simulink model "a3e2"  (R2020a)
settings: Solver=FixedStepAuto  StartTime=0.0  StopTime=40000  FixedStep=0.01  RelTol=1e-3
undefined symbols (not defined in the file): DiscIntNeverNeededParam
libraries: sldvlib x17
settings Model: EnablePacing=on  PacingRate=2  Creator=mumun  LastModifiedBy=mumun
settings ConfigComp: DVMode=PropertyProving  DVMaxProcessTime=10000000000  DVTestSuiteOptimization=Auto  DVDetectOutOfBounds=on

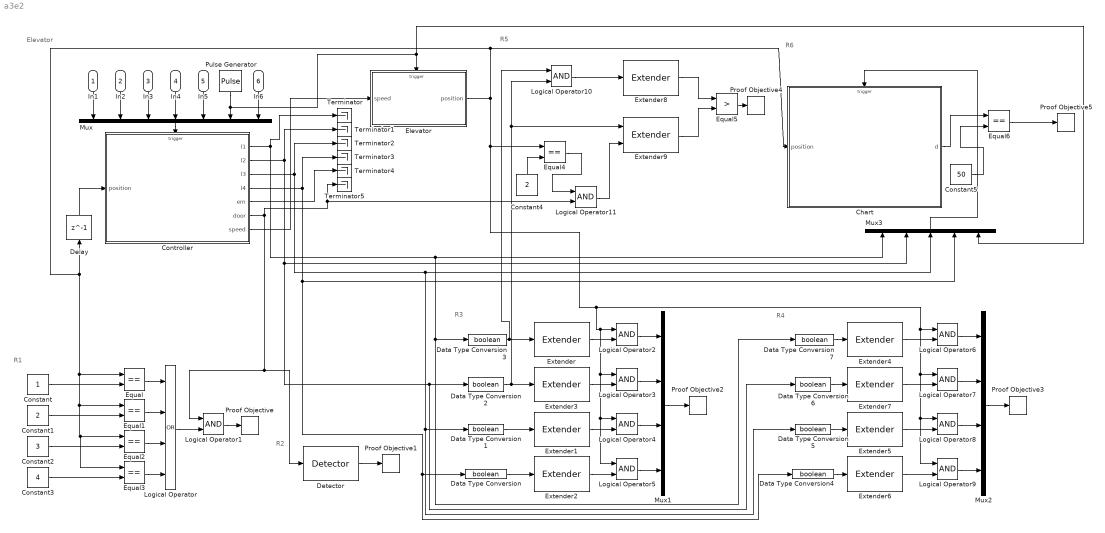
== system a3e2 ==
  note: R6
  note: R5
  note: R4
  note: Elevator
  note: R3
  note: R2
  note: R1
  In1 : Inport
  In2 : Inport  Port=2
  In3 : Inport  Port=3
  In4 : Inport  Port=4
  In5 : Inport  Port=5
  In6 : Inport  Port=6
  Chart : Stateflow chart  TreatAsAtomicUnit=on
  Constant : Constant
  Constant1 : Constant  Value=2
  Constant2 : Constant  Value=3
  Constant3 : Constant  Value=4
  Constant4 : Constant  Value=2
  Constant5 : Constant  Value=50
  Controller : Stateflow chart  TreatAsAtomicUnit=on
  Data Type Conversion{,1..7} (8 alike) : DataTypeConversion  OutDataTypeStr=boolean
  Delay : Delay  DelayLength=1  DelayLengthUpperLimit=2  InputProcessing=Columns as channels (frame based)  SampleTime=1
  Detector : sldvlib/Temporal Operators/Detector  reset=off  typ=Synchronized  in_hold=5  delay=1  out_hold=3
      settings: SourceProductBaseCode=SL
  Elevator : Stateflow chart  TreatAsAtomicUnit=on
  Equal{,1..4,6} (6 alike) : RelationalOperator  Operator===  OutDataTypeStr=boolean  RndMeth=Simplest
  Equal5 : RelationalOperator  Operator=>  OutDataTypeStr=boolean  RndMeth=Simplest
  Extender{,1..3} (4 alike) : sldvlib/Temporal Operators/Extender  reset=off  ext_type=Infinite  out_hold=5
      settings: SourceProductBaseCode=SL
  Extender{4..7} (4 alike) : sldvlib/Temporal Operators/Extender  reset=off  ext_type=Finite  out_hold=5
      settings: SourceProductBaseCode=SL
  Extender8 : sldvlib/Temporal Operators/Extender  reset=off  ext_type=Infinite  out_hold=3
      settings: SourceProductBaseCode=SL
  Extender9 : sldvlib/Temporal Operators/Extender  reset=on  ext_type=Infinite  out_hold=3
      settings: SourceProductBaseCode=SL
  Logical Operator : Logic  Operator=OR  Inputs=4  AllPortsSameDT=off  OutDataTypeStr=boolean
  Logical Operator{1..11} (11 alike) : Logic  AllPortsSameDT=off  OutDataTypeStr=boolean
  Mux : Mux  Inputs=7
  Mux1 : Mux
  Mux2 : Mux
  Mux3 : Mux  Inputs=5
  Proof Objective{,1..5} (6 alike) : sldvlib/Objectives and Constraints/Proof Objective  enabled=on  customAVTBlockType=Proof Objective  intervals=true  dispValues=on  outEnabled=off  enableStopSim=off
      settings: AttributesFormatString=%<intervals>  SourceProductBaseCode=SL
  Pulse Generator : DiscretePulseGenerator  PulseType=Time based  Period=1  PulseWidth=99  PhaseDelay=1
  Terminator{,1..5} (6 alike) : Terminator
  wires:
  In1/1 -> Mux/1
  In2/1 -> Mux/2
  In3/1 -> Mux/3
  In4/1 -> Mux/4
  In5/1 -> Mux/5
  Pulse Generator/1 -> Elevator/Trigger, Mux3/5, Mux/6
  Mux/1 -> Controller/Trigger
  In6/1 -> Mux/7
  Controller/5(em) -> Terminator4/1
  Controller/7(speed) -> Elevator/1(speed)
  Delay/1 -> Controller/1(position)
  Controller/1(l1) -> Terminator/1, Mux3/1, Data Type Conversion3/1, Data Type Conversion7/1
  Controller/2(l2) -> Terminator1/1, Mux3/2, Data Type Conversion6/1, Data Type Conversion2/1
  Controller/3(l3) -> Terminator2/1, Mux3/3, Data Type Conversion5/1, Data Type Conversion1/1
  Controller/4(l4) -> Terminator3/1, Mux3/4, Data Type Conversion4/1, Data Type Conversion/1
  Controller/6(door) -> Logical Operator11/2, Terminator5/1, Logical Operator1/1, Detector/1
  Detector/1 -> Proof Objective1/1
  Extender/1 -> Logical Operator2/2
  Extender1/1 -> Logical Operator4/2
  Extender3/1 -> Logical Operator3/2
  Extender2/1 -> Logical Operator5/2
  Logical Operator2/1 -> Mux1/1
  Logical Operator3/1 -> Mux1/2
  Logical Operator4/1 -> Mux1/3
  Logical Operator5/1 -> Mux1/4
  Mux1/1 -> Proof Objective2/1
  Data Type Conversion/1 -> Extender2/1
  Data Type Conversion1/1 -> Extender1/1
  Data Type Conversion2/1 -> Extender3/1, Extender9/1, Logical Operator10/2
  Data Type Conversion3/1 -> Logical Operator10/1, Extender/1
  Constant/1 -> Equal/2
  Constant1/1 -> Equal1/2
  Constant3/1 -> Equal3/2
  Constant2/1 -> Equal2/2
  Equal/1 -> Logical Operator/1
  Equal1/1 -> Logical Operator/2
  Equal2/1 -> Logical Operator/3
  Equal3/1 -> Logical Operator/4
  Logical Operator/1 -> Logical Operator1/2
  Logical Operator1/1 -> Proof Objective/1
  Extender5/1 -> Logical Operator8/2
  Extender4/1 -> Logical Operator6/2
  Data Type Conversion7/1 -> Extender4/1
  Logical Operator9/1 -> Mux2/4
  Logical Operator8/1 -> Mux2/3
  Mux2/1 -> Proof Objective3/1
  Logical Operator6/1 -> Mux2/1
  Extender7/1 -> Logical Operator7/2
  Data Type Conversion6/1 -> Extender7/1
  Data Type Conversion5/1 -> Extender5/1
  Elevator/1(position) -> Equal3/1, Equal2/1, Equal1/1, Equal/1, Delay/1, Chart/1(position), Logical Operator5/1, Logical Operator4/1, Logical Operator3/1, Logical Operator2/1, Logical Operator9/1, Logical Operator8/1, Logical Operator7/1, Logical Operator6/1, Equal4/1
  Logical Operator7/1 -> Mux2/2
  Extender6/1 -> Logical Operator9/2
  Data Type Conversion4/1 -> Extender6/1
  Logical Operator10/1 -> Extender8/1
  Constant4/1 -> Equal4/2
  Equal4/1 -> Logical Operator11/1
  Logical Operator11/1 -> Extender9/2
  Extender9/1 -> Equal5/2
  Extender8/1 -> Equal5/1
  Equal5/1 -> Proof Objective4/1
  Mux3/1 -> Chart/Trigger
  Constant5/1 -> Equal6/2
  Chart/1(d) -> Equal6/1
  Equal6/1 -> Proof Objective5/1

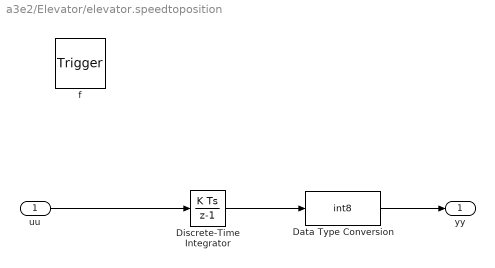
== system a3e2/Elevator/elevator.speedtoposition ==
  uu : Inport  OutDataTypeStr=double  PortDimensions=1
  f : TriggerPort  TriggerType=function-call  VariantControl=(inherit)
      settings: CopyFcn=Stateflow.SLINSF.SimulinkMan.removeBlockPreDeleteFcn  PreDeleteFcn=Stateflow.SLINSF.SimulinkMan.unsafePredeleteFcn
  Data Type Conversion : DataTypeConversion  OutDataTypeStr=int8  RndMeth=Round
  Discrete-Time Integrator : DiscreteIntegrator  InitialCondition=1  SampleTime=-1  LimitOutput=on  UpperSaturationLimit=4  LowerSaturationLimit=1  ICPrevOutput=DiscIntNeverNeededParam  ICPrevScaledInput=DiscIntNeverNeededParam
  yy : Outport
  wires:
  uu/1 -> Discrete-Time Integrator/1
  Discrete-Time Integrator/1 -> Data Type Conversion/1
  Data Type Conversion/1 -> yy/1

== stateflow chart a3e2/Elevator ==
  state elevator
    en, du: position=speedtoposition(speed)
    state yy = speedtoposition(uu) [function]
  (default) -> elevator
  data: uu function_input double size=1; yy function_output; speed input; position output
  events: pulse input EITHER_EDGE_EVENT

== stateflow chart a3e2/Chart ==
  state R6
    en:time=0; floor1=0; floor2=0; floor3=0; floor4=0; d=0;
    on pulse: time_counter();
    on one: floor1= time;
    on two: floor2= time;
    on three: floor3= time;
    on four: floor4= time;
    state floor3
      en: d=time-floor3;
    state floor2
      en: d=time-floor2;
    state floor4
      en: d=time-floor4;
    state floor1
      en: d=time-floor1;
    floor3 -> floor2 [order 2] : [position==2]
    floor2 -> floor3 [order 1] : [position==3]
    floor2 -> floor1 [order 2] : [position==1]
    floor1 -> floor2 : [position==2]
    floor4 -> floor3 : [position==3]
    floor3 -> floor4 [order 1] : [position==4]
    (default) -> floor1
  (default) -> R6
  data: time local double; floor1 local double; floor2 local double; floor3 local double; floor4 local double; d output double; position input
  events: one input RISING_EDGE_EVENT; two input RISING_EDGE_EVENT; three input RISING_EDGE_EVENT; four input RISING_EDGE_EVENT; pulse input EITHER_EDGE_EVENT
  function time_counter:
    | function time_counter
    | time =(time+1);
    | 
    | end

== stateflow chart a3e2/Controller ==
  settings: executeAtInitialization=1
  state controller
    en: em=0; go1=0; go2=0; go3=0; go4=0; door=0;t=0; l1=0;l2=0;l3=0;l4=0;
    on Floor_1:  go1=1;l1=1;
    on Floor_2:  go2=1;l2=1;
    on Floor_3:  go3=1;l3=1;
    on Floor_4:  go4=1;l4=1;
    on emergency: em=1;
    on restart: em=0;
    en, du: controllerlogic();
    state floor3
      state closed
        du:door=0;
      state open
        en,du: door=1;l3=0;
        en,du: t=elapsed(sec);
        exit: door=0;go3=0;
      (default) -> controller.floor3.closed
      controller.floor3.open -> controller.floor3.closed : [t>=5]
      controller.floor3.closed -> controller.floor3.open : [l3==1]
    state floor2
      state closed
        du:door=0;
      state open
        en,du: door=1;l2=0;
        en,du: t=elapsed(sec);
        exit: door=0;go2=0;
      (default) -> controller.floor2.closed
      controller.floor2.open -> controller.floor2.closed : [t>=5]
      controller.floor2.closed -> controller.floor2.open : [l2==1]
    state floor4
      state closed
        du:door=0;
      state open
        en,du: door=1;l4=0;
        en,du: t=elapsed(sec);
        exit: door=0;go4=0;
      (default) -> controller.floor4.closed
      controller.floor4.open -> controller.floor4.closed : [t>=5]
      controller.floor4.closed -> controller.floor4.open : [l4==1]
    state floor1
      state closed
        du:door=0;
      state open
        en,du: door=1;l1=0;
        en,du: t=elapsed(sec);
        exit: door=0;go1=0;
      (default) -> controller.floor1.closed
      controller.floor1.open -> controller.floor1.closed : [t>=5]
      controller.floor1.closed -> controller.floor1.open : [l1==1]
    floor3 -> floor2 [order 2] : [position==2]
    floor2 -> floor3 [order 1] : [position==3]
    floor2 -> floor1 [order 2] : [position==1]
    floor1 -> floor2 : [position==2]
    floor4 -> floor3 : [position==3]
    floor3 -> floor4 [order 1] : [position==4]
    (default) -> floor1
  (default) -> controller
  data: l1 output double size=1; l2 output double size=1; l3 output double size=1; l4 output double size=1; em output double size=1; door output boolean size=1; speed output double size=1; position input double size=1; t local double size=1; go1 local double size=1; go2 local double size=1; go3 local double size=1; go4 local double size=1
  events: Floor_1 input RISING_EDGE_EVENT; Floor_2 input RISING_EDGE_EVENT; Floor_3 input RISING_EDGE_EVENT; Floor_4 input RISING_EDGE_EVENT; emergency input RISING_EDGE_EVENT; pulse input EITHER_EDGE_EVENT; restart input RISING_EDGE_EVENT
  function controllerlogic:
    | function controllerlogic
    | max_speed= 0.2;
    | current_floor= round(position);
    | % destination_floor= 1;
    | % go=1;
    | 
    | if em == 0 && go1==1
    |     destination_floor= 1;
    |         if destination_floor-current_floor==0
    |             speed= 0;
    |             go1=0;
    |         elseif destination_floor-current_floor> 0
    |             speed= max_speed;          
    |         elseif destination_floor-(current_floor+1)< 0
    |             speed= -1*max_speed;
    |         end       
    | elseif em == 0 && go2==1
    |     destination_floor= 2;
    |         if destination_floor-current_floor==0
    |             speed= 0;
    |             go2=0;
    |         elseif destination_floor-current_floor> 0
    |             speed= max_speed;          
    |         elseif destination_floor-(current_floor+1)< 0
    |             speed= -1*max_speed;
    |         end
    | elseif em == 0 && go3==1
    |     destination_floor= 3;
    |         if destination_floor-current_floor==0
    |             speed= 0;
    |             go3=0;
    |         elseif destination_floor-current_floor> 0
    |             speed= max_speed;          
    |         elseif destination_floor-(current_floor+1)< 0
    |             speed= -1*max_speed;
    |         end
    | elseif em == 0 && go4==1
    |     destination_floor= 4;
    |         if destination_floor-current_floor==0
    |             speed= 0;
    |             go4=0;
    |         elseif destination_floor-current_floor> 0
    |             speed= max_speed;          
    |         elseif destination_floor-(current_floor+1)< 0
    |             speed= -1*max_speed;
    |         end        
    | elseif em == 1
    |     destination_floor= 1;
    |         if destination_floor-current_floor==0
    |             speed= 0;
    |             go2=0;
    |             go3=0;
    |             go4=0;
    |             l2=0;
    |             l3=0;
    |             l4=0;
    |         elseif destination_floor-current_floor> 0
    |             speed= max_speed;
    |         elseif destination_floor-(current_floor+1)< 0
    |             speed= -1*max_speed;
    |         end
    | end
    | end
